simulink subsystem "guiado3"  (R2021b)
settings: Solver=VariableStepAuto  StartTime=0.0  StopTime=10.0  RelTol=1e-3
values from neighbouring files (symbols this model uses):
  fp = [t1;t2;t3]    [creacionestructurasborrador.m]    (also in flight_plan.m = [sid,wps,iap]; flight_plan_eval.m = [t1;tabla2;t3]; flight_plan_old.m = [sid,wps,iap]; flight_plan_struct.m = [t1;tabla2;t3])
libraries: simulink x6
settings Model: Creator=verti  LastModifiedBy=verti

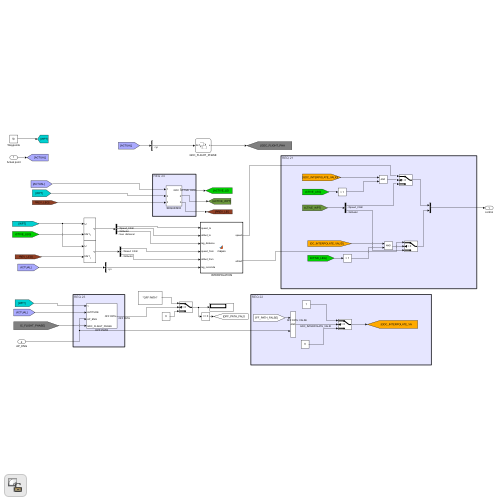
[thumbnail: Simulink's stored preview of the top-level diagram]
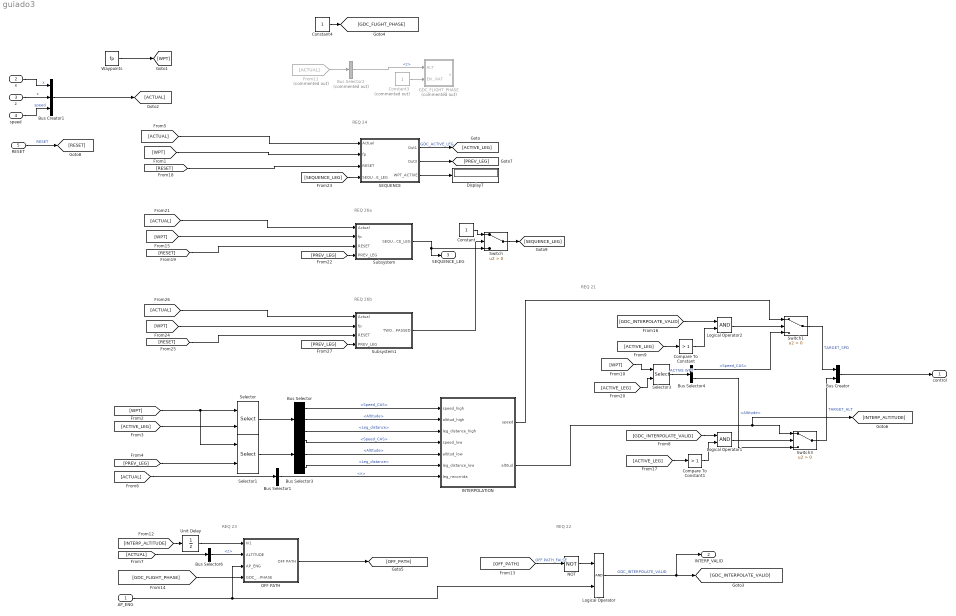
== system guiado3 ==
  note: REQ 24
  note: REQ 22
  note: REQ 23
  note: REQ 21
  note: REQ 26a
  note: REQ 26b
  AP_ENG : Inport
  x : Inport  Port=2
  z : Inport  Port=3
  speed : Inport  Port=4
  RESET : Inport  Port=5
  Bus Creator : BusCreator  Inputs=2
  Bus Creator1 : BusCreator  Inputs=3
  Bus Selector : BusSelector  OutputSignals=Speed_CAS,Altitude,Leg_distance
  Bus Selector1 : BusSelector  OutputSignals=x
  Bus Selector2 : BusSelector  Commented=on  OutputSignals=z
  Bus Selector3 : BusSelector  OutputSignals=Speed_CAS,Altitude,Leg_distance
  Bus Selector4 : BusSelector  OutputSignals=Speed_CAS,Altitude
  Bus Selector6 : BusSelector  OutputSignals=z
  Compare To Constant : simulink/Logic and Bit Operations/Compare To Constant  relop=>  const=1  OutDataTypeStr=boolean
  Compare To Constant1 : simulink/Logic and Bit Operations/Compare To Constant  relop=>  const=1  OutDataTypeStr=boolean
  Constant : Constant
  Constant3 : Constant  Commented=on
  Constant4 : Constant
  Display7 : Display
  From11 : From  Commented=on  GotoTag=ACTUAL
  GDC_FLIGHT_PHASE : Stateflow chart  Commented=on  TreatAsAtomicUnit=on
  INTERPOLATION : MATLAB Function  TreatAsAtomicUnit=on
  Logical Operator : Logic  AllPortsSameDT=off  OutDataTypeStr=boolean
  Logical Operator1 : Logic  AllPortsSameDT=off  OutDataTypeStr=boolean
  Logical Operator2 : Logic  AllPortsSameDT=off  OutDataTypeStr=boolean
  NOT : Logic  Operator=NOT  IconShape=distinctive  AllPortsSameDT=off  OutDataTypeStr=boolean
  OFF PATH : Subsystem
  SEQUENCE : Subsystem
  Selector : Selector  InputPortWidth=12  IndexOptions=Index vector (port)  Indices=[1 3]  OutputSizes=1
  Selector1 : Selector  InputPortWidth=12  IndexOptions=Index vector (port)  Indices=[1 3]  OutputSizes=1
  Selector3 : Selector  InputPortWidth=12  IndexOptions=Index vector (port)  Indices=[1 3]  OutputSizes=1
  Subsystem : Subsystem
  Subsystem1 : Subsystem
  Switch : Switch  Criteria=u2 > Threshold
  Switch1 : Switch  Criteria=u2 > Threshold
  Switch3 : Switch  Criteria=u2 > Threshold
  Unit Delay : UnitDelay  SampleTime=-1  HasFrameUpgradeWarning=on
  Waypoints : Constant  Value=fp  OutDataTypeStr=Bus: BUS_FP
  control : Outport
  INTERP_VALID : Outport  Port=2
  SEQUENCE_LEG : Outport  Port=3
  wires:
  NOT/1 -> Logical Operator/1
  [INTERP_ALTITUDE] -> Unit Delay/1
  Unit Delay/1 -> OFF PATH/1(In1)
  SEQUENCE/3(WPT_ACTIVE) -> Display7/1
  [PREV_LEG] -> Selector1/2
  Bus Selector3/3 -> INTERPOLATION/6(leg_distance_low)  "<Leg_distance>"
  [ACTIVE_LEG] -> Selector/2
  Selector3/1 -> Bus Selector4/1  "ACTIVE WPT"
  [ACTIVE_LEG] -> Selector3/2
  [WPT] -> Selector3/1
  Logical Operator2/1 -> Switch1/2
  Bus Selector3/2 -> INTERPOLATION/5(altitud_low)  "<Altitude>"
  Bus Selector/1 -> INTERPOLATION/1(speed_high)  "<Speed_CAS>"
  Bus Selector/3 -> INTERPOLATION/3(leg_distance_high)  "<Leg_distance>"
  [ACTIVE_LEG] -> Compare To Constant/1
  Switch3/1 -> Bus Creator/2  "TARGET_ALT"
  Bus Creator/1 -> control/1
  Compare To Constant/1 -> Logical Operator2/2
  Bus Selector4/1 -> Switch1/3  "<Speed_CAS>"
  [WPT] -> Selector1/1, Selector/1
  Selector1/1 -> Bus Selector3/1
  [ACTIVE_LEG] -> Compare To Constant1/1
  INTERPOLATION/2(altitud) -> Switch3/1, [INTERP_ALTITUDE]
  Compare To Constant1/1 -> Logical Operator1/2
  [GDC_FLIGHT_PHASE] -> OFF PATH/4(GDC_FLIGHT_PHASE)
  Selector/1 -> Bus Selector/1
  From11/1 -> Bus Selector2/1
  Bus Selector3/1 -> INTERPOLATION/4(speed_low)  "<Speed_CAS>"
  SEQUENCE/2(Out3) -> [PREV_LEG]
  [GDC_INTERPOLATE_VALID] -> Logical Operator1/1
  [OFF_PATH] -> NOT/1  "OFF PATH_FALSE"
  Bus Selector/2 -> INTERPOLATION/2(altitud_high)  "<Altitude>"
  Logical Operator1/1 -> Switch3/2
  Switch1/1 -> Bus Creator/1  "TARGET_SPD"
  Bus Selector4/2 -> Switch3/3  "<Altitude>"
  [ACTUAL] -> Bus Selector1/1
  [ACTUAL] -> SEQUENCE/1(Actual)
  Waypoints/1 -> [WPT]
  SEQUENCE/1(Out1) -> [ACTIVE_LEG]  "GDC_ACTIVE_LEG"
  AP_ENG/1 -> OFF PATH/3(AP_ENG), Logical Operator/2
  Bus Selector2/1 -> GDC_FLIGHT_PHASE/1(ALT)  "<z>"
  Logical Operator/1 -> INTERP_VALID/1, [GDC_INTERPOLATE_VALID]  "GDC_INTERPOLATE_VALID"
  INTERPOLATION/1(speed) -> Switch1/1
  [GDC_INTERPOLATE_VALID] -> Logical Operator2/1
  [WPT] -> SEQUENCE/2(fp)
  Bus Selector1/1 -> INTERPOLATION/7(leg_recorrida)  "<x>"
  Bus Creator1/1 -> [ACTUAL]
  z/1 -> Bus Creator1/2  "z"
  x/1 -> Bus Creator1/1  "x"
  speed/1 -> Bus Creator1/3  "speed"
  Constant3/1 -> GDC_FLIGHT_PHASE/2(ENG_RAT)
  Constant4/1 -> [GDC_FLIGHT_PHASE]
  [ACTUAL] -> Bus Selector6/1
  Bus Selector6/1 -> OFF PATH/2(ALTITUDE)  "<z>"
  RESET/1 -> [RESET]  "RESET"
  [RESET] -> SEQUENCE/3(RESET)
  OFF PATH/1(OFF PATH) -> [OFF_PATH]
  [RESET] -> Subsystem/3(RESET)
  [WPT] -> Subsystem/2(fp)
  [ACTUAL] -> Subsystem/1(Actual)
  [PREV_LEG] -> Subsystem/4(PREV_LEG)
  Subsystem/1(SEQUENCE_LEG) -> SEQUENCE_LEG/1, Switch/3
  [SEQUENCE_LEG] -> SEQUENCE/4(SEQUENCE_LEG)
  Subsystem1/1(TWO_WP_PASSED) -> Switch/2
  [PREV_LEG] -> Subsystem1/4(PREV_LEG)
  [ACTUAL] -> Subsystem1/1(Actual)
  [WPT] -> Subsystem1/2(fp)
  [RESET] -> Subsystem1/3(RESET)
  Switch/1 -> [SEQUENCE_LEG]
  Constant/1 -> Switch/1

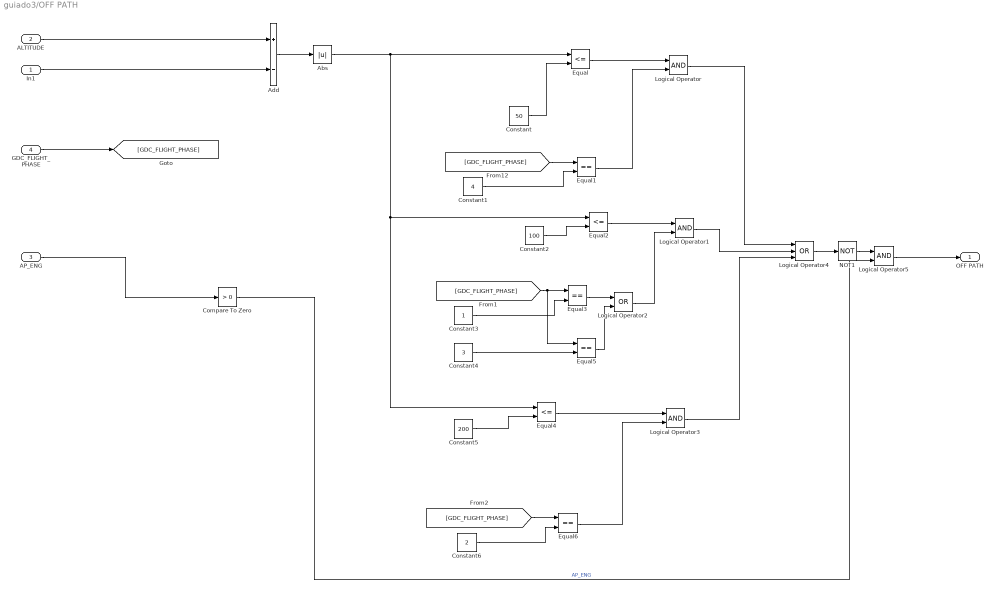
== system guiado3/OFF PATH ==
  In1 : Inport
  ALTITUDE : Inport  Port=2
  AP_ENG : Inport  Port=3
  GDC_FLIGHT_PHASE : Inport  Port=4
  Abs : Abs
  Add : Sum  Inputs=+-
  Compare To Zero : simulink/Logic and Bit Operations/Compare To Zero  relop=>  OutDataTypeStr=boolean
  Constant : Constant  Value=50
  Constant1 : Constant  Value=4
  Constant2 : Constant  Value=100
  Constant3 : Constant
  Constant4 : Constant  Value=3
  Constant5 : Constant  Value=200
  Constant6 : Constant  Value=2
  Equal : RelationalOperator  Operator=<=  OutDataTypeStr=boolean  RndMeth=Simplest
  Equal{1,3,5..6} (4 alike) : RelationalOperator  Operator===  OutDataTypeStr=boolean  RndMeth=Simplest
  Equal2 : RelationalOperator  Operator=<=  OutDataTypeStr=boolean  RndMeth=Simplest
  Equal4 : RelationalOperator  Operator=<=  OutDataTypeStr=boolean  RndMeth=Simplest
  Logical Operator{,1,3,5} (4 alike) : Logic  AllPortsSameDT=off  OutDataTypeStr=boolean
  Logical Operator2 : Logic  Operator=OR  AllPortsSameDT=off  OutDataTypeStr=boolean
  Logical Operator4 : Logic  Operator=OR  Inputs=3  AllPortsSameDT=off  OutDataTypeStr=boolean
  NOT1 : Logic  Operator=NOT  IconShape=distinctive  AllPortsSameDT=off  OutDataTypeStr=boolean
  OFF PATH : Outport
  wires:
  NOT1/1 -> Logical Operator5/1
  Logical Operator5/1 -> OFF PATH/1
  AP_ENG/1 -> Compare To Zero/1
  Compare To Zero/1 -> Logical Operator5/2  "AP_ENG"
  Add/1 -> Abs/1
  Constant/1 -> Equal/2
  Abs/1 -> Equal4/1, Equal2/1, Equal/1
  [GDC_FLIGHT_PHASE] -> Equal1/1
  Constant1/1 -> Equal1/2
  Equal1/1 -> Logical Operator/2
  Equal/1 -> Logical Operator/1
  Constant2/1 -> Equal2/2
  Constant3/1 -> Equal3/2
  [GDC_FLIGHT_PHASE] -> Equal5/1, Equal3/1
  Equal2/1 -> Logical Operator1/1
  Equal3/1 -> Logical Operator2/1
  Constant4/1 -> Equal5/2
  Equal5/1 -> Logical Operator2/2
  Logical Operator2/1 -> Logical Operator1/2
  Constant5/1 -> Equal4/2
  Constant6/1 -> Equal6/2
  [GDC_FLIGHT_PHASE] -> Equal6/1
  Equal6/1 -> Logical Operator3/2
  Equal4/1 -> Logical Operator3/1
  Logical Operator/1 -> Logical Operator4/1
  Logical Operator1/1 -> Logical Operator4/2
  Logical Operator3/1 -> Logical Operator4/3
  Logical Operator4/1 -> NOT1/1
  In1/1 -> Add/2
  GDC_FLIGHT_PHASE/1 -> [GDC_FLIGHT_PHASE]
  ALTITUDE/1 -> Add/1

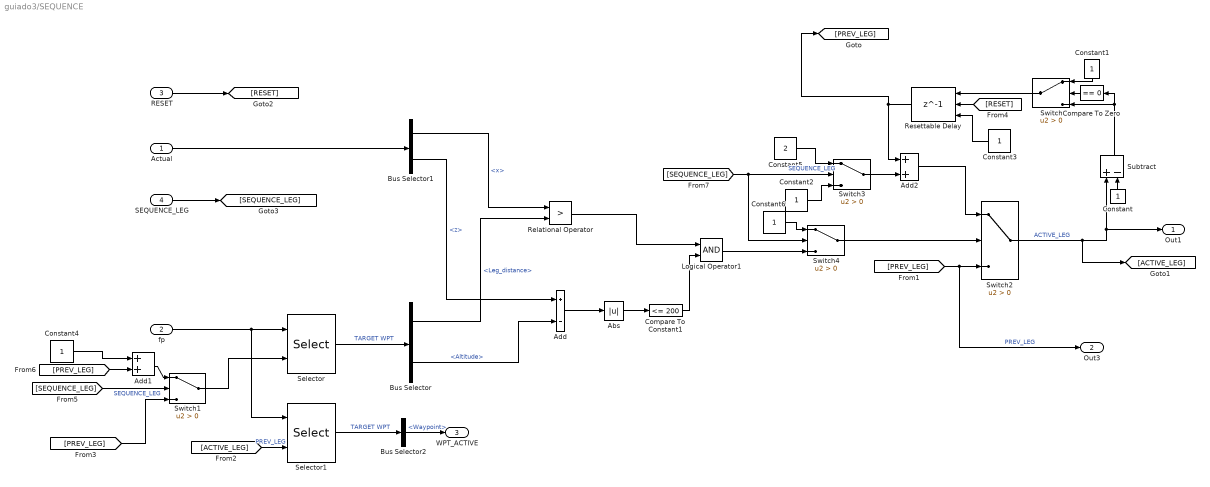
== system guiado3/SEQUENCE ==
  Actual : Inport
  fp : Inport  Port=2
  RESET : Inport  Port=3
  SEQUENCE_LEG : Inport  Port=4
  Abs : Abs
  Add : Sum  Inputs=+-
  Add1 : Sum
  Add2 : Sum
  Bus Selector : BusSelector  OutputSignals=Leg_distance,Altitude
  Bus Selector1 : BusSelector  OutputSignals=x,z
  Bus Selector2 : BusSelector  OutputSignals=Waypoint
  Compare To Constant1 : simulink/Logic and Bit Operations/Compare To Constant  relop=<=  const=200  OutDataTypeStr=boolean
  Compare To Zero : simulink/Logic and Bit Operations/Compare To Zero  relop===  OutDataTypeStr=boolean
  Constant{,1..4,6} (6 alike) : Constant
  Constant5 : Constant  Value=2
  Logical Operator1 : Logic  AllPortsSameDT=off  OutDataTypeStr=boolean
  Relational Operator : RelationalOperator  Operator=>  OutDataTypeStr=boolean  RndMeth=Simplest
  Resettable Delay : Delay  DelayLength=1  InitialConditionSource=Input port  ExternalReset=Rising
      settings: InputPortMap=u0,r5,p4
  Selector : Selector  InputPortWidth=12  IndexOptions=Index vector (port)  Indices=[1 3]  OutputSizes=1
  Selector1 : Selector  InputPortWidth=12  IndexOptions=Index vector (port)  Indices=[1 3]  OutputSizes=1
  Subtract : Sum  Inputs=+-
  Switch{,1..4} (5 alike) : Switch  Criteria=u2 > Threshold
  Out1 : Outport
  Out3 : Outport  Port=2
  WPT_ACTIVE : Outport  Port=3
  wires:
  Constant6/1 -> Switch4/1
  Switch4/1 -> Switch2/2
  Constant2/1 -> Switch3/3
  Switch3/1 -> Add2/2
  [SEQUENCE_LEG] -> Switch3/2, Switch4/2  "SEQUENCE_LEG"
  Constant5/1 -> Switch3/1
  Switch1/1 -> Selector/2
  Add1/1 -> Switch1/1
  [PREV_LEG] -> Add1/2
  Constant4/1 -> Add1/1
  [SEQUENCE_LEG] -> Switch1/2  "SEQUENCE_LEG"
  Logical Operator1/1 -> Switch4/3
  SEQUENCE_LEG/1 -> [SEQUENCE_LEG]
  [RESET] -> Resettable Delay/2
  RESET/1 -> [RESET]
  Constant3/1 -> Resettable Delay/3
  [PREV_LEG] -> Out3/1, Switch2/3  "PREV_LEG"
  Selector/1 -> Bus Selector/1  "TARGET WPT"
  fp/1 -> Selector1/1, Selector/1
  Add/1 -> Abs/1
  Add2/1 -> Switch2/1
  Compare To Constant1/1 -> Logical Operator1/2
  Actual/1 -> Bus Selector1/1
  Bus Selector1/2 -> Add/1  "<z>"
  Relational Operator/1 -> Logical Operator1/1
  Bus Selector/1 -> Relational Operator/2  "<Leg_distance>"
  Resettable Delay/1 -> Add2/1, [PREV_LEG]
  Abs/1 -> Compare To Constant1/1
  Bus Selector1/1 -> Relational Operator/1  "<x>"
  Bus Selector/2 -> Add/2  "<Altitude>"
  [PREV_LEG] -> Switch1/3
  Subtract/1 -> Switch/3, Compare To Zero/1
  Constant/1 -> Subtract/2
  Compare To Zero/1 -> Switch/2
  Switch/1 -> Resettable Delay/1
  Constant1/1 -> Switch/1
  Switch2/1 -> [ACTIVE_LEG], Out1/1, Subtract/1  "ACTIVE_LEG"
  [ACTIVE_LEG] -> Selector1/2  "PREV_LEG"
  Selector1/1 -> Bus Selector2/1  "TARGET WPT"
  Bus Selector2/1 -> WPT_ACTIVE/1  "<Waypoint>"

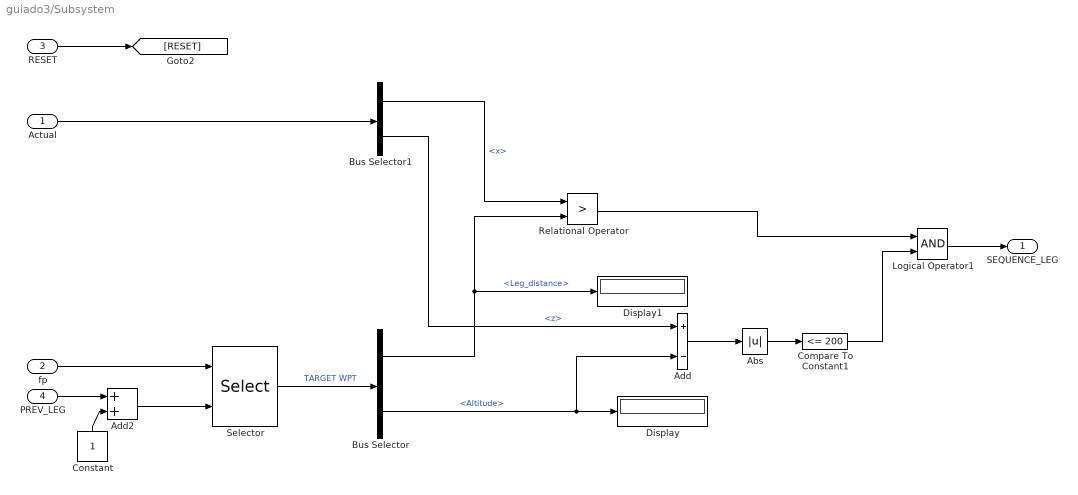
== system guiado3/Subsystem ==
  Actual : Inport
  fp : Inport  Port=2
  RESET : Inport  Port=3
  PREV_LEG : Inport  Port=4
  Abs : Abs
  Add : Sum  Inputs=+-
  Add2 : Sum
  Bus Selector : BusSelector  OutputSignals=Leg_distance,Altitude
  Bus Selector1 : BusSelector  OutputSignals=x,z
  Compare To Constant1 : simulink/Logic and Bit Operations/Compare To Constant  relop=<=  const=200  OutDataTypeStr=boolean
  Constant : Constant
  Display : Display
  Display1 : Display
  Logical Operator1 : Logic  AllPortsSameDT=off  OutDataTypeStr=boolean
  Relational Operator : RelationalOperator  Operator=>  OutDataTypeStr=boolean  RndMeth=Simplest
  Selector : Selector  InputPortWidth=12  IndexOptions=Index vector (port)  Indices=[1 3]  OutputSizes=1
  SEQUENCE_LEG : Outport
  wires:
  Logical Operator1/1 -> SEQUENCE_LEG/1
  Constant/1 -> Add2/2
  PREV_LEG/1 -> Add2/1
  Bus Selector1/1 -> Relational Operator/1  "<x>"
  Abs/1 -> Compare To Constant1/1
  Actual/1 -> Bus Selector1/1
  RESET/1 -> [RESET]
  Selector/1 -> Bus Selector/1  "TARGET WPT"
  Compare To Constant1/1 -> Logical Operator1/2
  Bus Selector1/2 -> Add/1  "<z>"
  Bus Selector/1 -> Relational Operator/2, Display1/1  "<Leg_distance>"
  Add2/1 -> Selector/2
  Bus Selector/2 -> Display/1, Add/2  "<Altitude>"
  fp/1 -> Selector/1
  Add/1 -> Abs/1
  Relational Operator/1 -> Logical Operator1/1

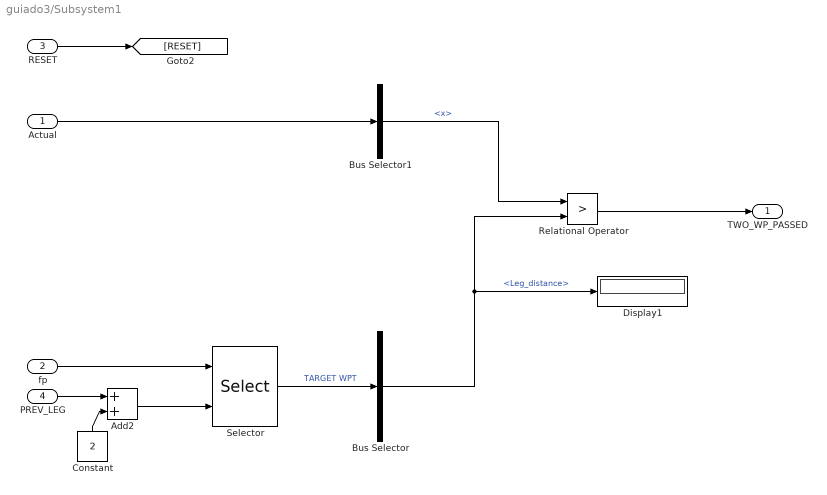
== system guiado3/Subsystem1 ==
  Actual : Inport
  fp : Inport  Port=2
  RESET : Inport  Port=3
  PREV_LEG : Inport  Port=4
  Add2 : Sum
  Bus Selector : BusSelector  OutputSignals=Leg_distance
  Bus Selector1 : BusSelector  OutputSignals=x
  Constant : Constant  Value=2
  Display1 : Display
  Relational Operator : RelationalOperator  Operator=>  OutDataTypeStr=boolean  RndMeth=Simplest
  Selector : Selector  InputPortWidth=12  IndexOptions=Index vector (port)  Indices=[1 3]  OutputSizes=1
  TWO_WP_PASSED : Outport
  wires:
  fp/1 -> Selector/1
  Add2/1 -> Selector/2
  Bus Selector/1 -> Display1/1, Relational Operator/2  "<Leg_distance>"
  Selector/1 -> Bus Selector/1  "TARGET WPT"
  RESET/1 -> [RESET]
  Actual/1 -> Bus Selector1/1
  Bus Selector1/1 -> Relational Operator/1  "<x>"
  PREV_LEG/1 -> Add2/1
  Constant/1 -> Add2/2
  Relational Operator/1 -> TWO_WP_PASSED/1

== stateflow chart guiado3/GDC_FLIGHT_PHASE ==
  state CRUISE
    entry:
    x==2;
  state CLIMB
    entry:
    x==1;
  state DESCEND
    entry:
    x==3;
  state APPROACH
    entry:
    x==4;
  (default) -> CLIMB
  DESCEND -> APPROACH : [ALT<2000]
  CLIMB -> CRUISE : [ALT>=CRZ_ALT]
  CRUISE -> DESCEND [order 2] : [(ALT<CRZ_ALT) & (ENG_RAT==IDLE)]
  CRUISE -> CLIMB [order 1] : [ALT<CRZ_ALT & (ENG_RAT==MTO | ENG_RAT==MCT | ENG_RAT==CLB)]
  data: ALT input; x output; CRZ_ALT constant double =30000; CLB constant double =2; MTO constant double =4; MCT local =3; IDLE constant double =1; ENG_RAT input

== matlab function guiado3/INTERPOLATION ==
  data: speed_high input; altitud_high input; leg_distance_high input; speed_low input; altitud_low input; leg_distance_low input; leg_recorrida input; speed output; altitud output
function [speed,altitud] = mapeo(speed_high,altitud_high,leg_distance_high,speed_low,altitud_low,leg_distance_low,leg_recorrida)

speed = (leg_recorrida-leg_distance_low) .* (speed_high - speed_low) ./ (leg_distance_high - leg_distance_low) + speed_low;
altitud = (leg_recorrida-leg_distance_low) .* (altitud_high - altitud_low) ./ (leg_distance_high- leg_distance_low) + altitud_low;

end
